simulink model "simulatePDcontrol"  (R2025a)
settings: Solver=VariableStepAuto  StartTime=0.0  StopTime=10.0  RelTol=1e-3
settings Model: Creator=doanb  LastModifiedBy=malvikabhardwaj

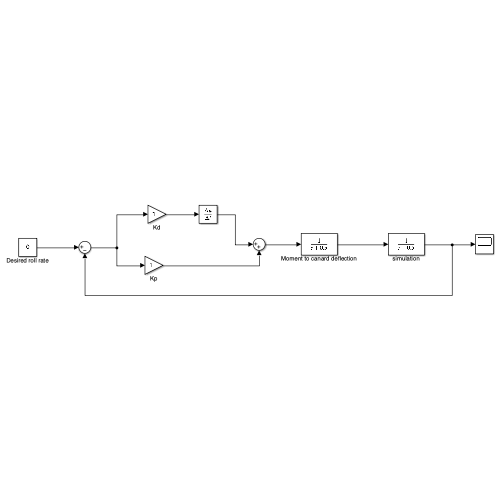
[thumbnail: Simulink's stored preview of the top-level diagram]
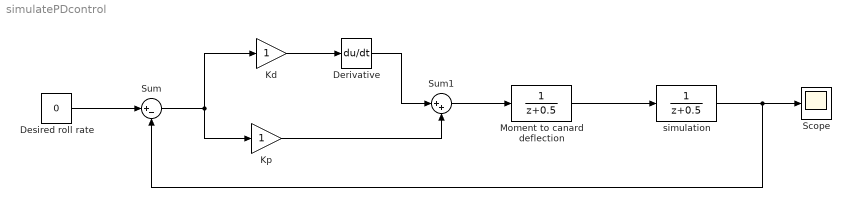
== system simulatePDcontrol ==
  Derivative : Derivative
  Desired roll rate : Constant  Value=0
  Kd : Gain
  Kp : Gain
  Moment to canard deflection : DiscreteTransferFcn
  Scope : Scope
  Sum : Sum  Inputs=|+-
  Sum1 : Sum  Inputs=|++
  simulation : DiscreteTransferFcn
  wires:
  Desired roll rate/1 -> Sum/1
  Sum/1 -> Kp/1, Kd/1
  Kd/1 -> Derivative/1
  Kp/1 -> Sum1/2
  Derivative/1 -> Sum1/1
  Sum1/1 -> Moment to canard deflection/1
  Moment to canard deflection/1 -> simulation/1
  simulation/1 -> Sum/2, Scope/1
